simulink model "pendule_inv_echant_etu"  (R2022b)
settings: Solver=VariableStepAuto  StartTime=0.0  StopTime=10.0  RelTol=1e-3
values from neighbouring files (symbols this model uses):
  g = 9.81    [simu_pendule_inv_capteur_etu.m]    (also in simu_pendule_inv_etu.m)
  K = [10 1]    [simu_pendule_inv_capteur_etu.m]    (also in simu_pendule_inv_etu.m = [30 10])
  l = 10    [simu_pendule_inv_capteur_etu.m]    (also in simu_pendule_inv_etu.m)
  ue = 0    [simu_pendule_inv_capteur_etu.m]    (also in simu_pendule_inv_etu.m)
  x0 = [pi/20 0]'    [simu_pendule_inv_capteur_etu.m]    (also in simu_pendule_inv_etu.m = [pi/10 0]')
  xe = [0 0]'    [simu_pendule_inv_capteur_etu.m]    (also in simu_pendule_inv_etu.m)
undefined symbols (not defined in the file or in its folder): delta_t, DiscIntNeverNeededParam
settings Model: Creator=marga  LastModifiedBy=marga

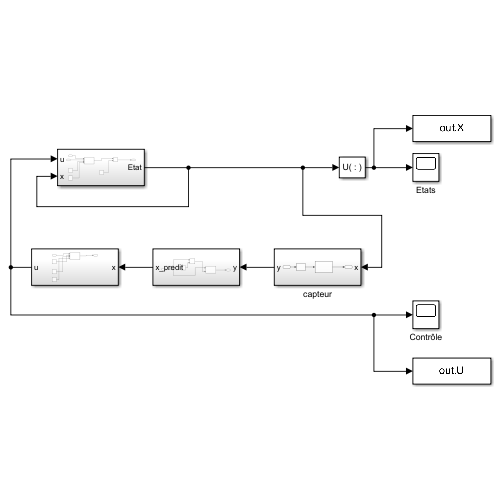
[thumbnail: Simulink's stored preview of the top-level diagram]
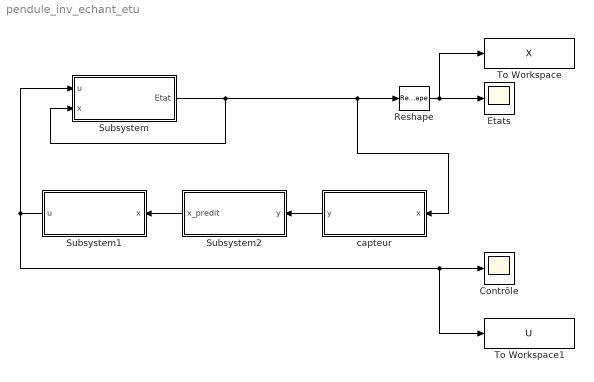
== system pendule_inv_echant_etu ==
  Contrôle : Scope
  Etats : Scope
  Reshape : Reshape
  Subsystem : Subsystem
  Subsystem1 : Subsystem
  Subsystem2 : Subsystem
  To Workspace : ToWorkspace  VariableName=X  SaveFormat=Timeseries  SampleTime=-1
  To Workspace1 : ToWorkspace  VariableName=U  SaveFormat=Timeseries  SampleTime=-1
  capteur : Subsystem
  wires:
  Subsystem2/1(x_predit) -> Subsystem1/1(x)
  capteur/1(y) -> Subsystem2/1(y)
  Reshape/1 -> To Workspace/1, Etats/1
  Subsystem/1(Etat) -> Subsystem/2(x), capteur/1(x), Reshape/1
  Subsystem1/1(u) -> Subsystem/1(u), To Workspace1/1, Contrôle/1

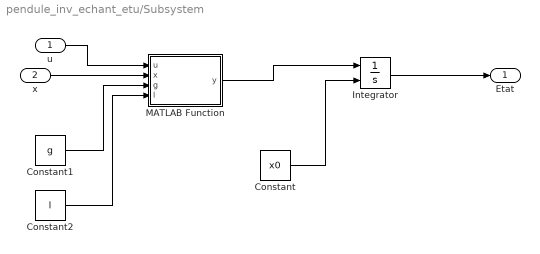
== system pendule_inv_echant_etu/Subsystem ==
  u : Inport
  x : Inport  Port=2
  Constant : Constant  Value=x0
  Constant1 : Constant  Value=g
  Constant2 : Constant  Value=l
  Integrator : Integrator  InitialConditionSource=external
  MATLAB Function : MATLAB Function  TreatAsAtomicUnit=on
  Etat : Outport
  wires:
  Constant/1 -> Integrator/2
  u/1 -> MATLAB Function/1(u)
  Integrator/1 -> Etat/1
  Constant1/1 -> MATLAB Function/3(g)
  Constant2/1 -> MATLAB Function/4(l)
  MATLAB Function/1(y) -> Integrator/1
  x/1 -> MATLAB Function/2(x)

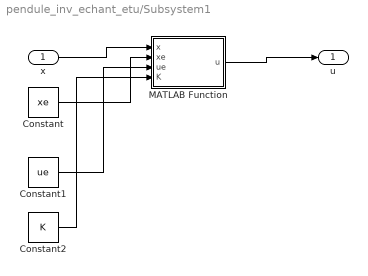
== system pendule_inv_echant_etu/Subsystem1 ==
  x : Inport
  Constant : Constant  Value=xe
  Constant1 : Constant  Value=ue
  Constant2 : Constant  Value=K  VectorParams1D=off
  MATLAB Function : MATLAB Function  TreatAsAtomicUnit=on
  u : Outport
  wires:
  x/1 -> MATLAB Function/1(x)
  MATLAB Function/1(u) -> u/1
  Constant/1 -> MATLAB Function/2(xe)
  Constant1/1 -> MATLAB Function/3(ue)
  Constant2/1 -> MATLAB Function/4(K)

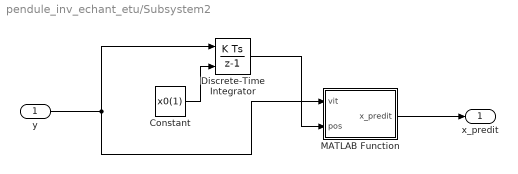
== system pendule_inv_echant_etu/Subsystem2 ==
  y : Inport
  Constant : Constant  Value=x0(1)
  Discrete-Time Integrator : DiscreteIntegrator  InitialConditionSource=external  SampleTime=delta_t  ICPrevOutput=DiscIntNeverNeededParam  ICPrevScaledInput=DiscIntNeverNeededParam
  MATLAB Function : MATLAB Function  TreatAsAtomicUnit=on
  x_predit : Outport
  wires:
  y/1 -> Discrete-Time Integrator/1, MATLAB Function/1(vit)
  Discrete-Time Integrator/1 -> MATLAB Function/2(pos)
  MATLAB Function/1(x_predit) -> x_predit/1
  Constant/1 -> Discrete-Time Integrator/2

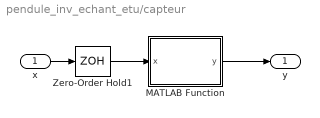
== system pendule_inv_echant_etu/capteur ==
  x : Inport
  MATLAB Function : MATLAB Function  TreatAsAtomicUnit=on
  Zero-Order Hold1 : ZeroOrderHold  SampleTime=delta_t
  y : Outport
  wires:
  x/1 -> Zero-Order Hold1/1
  MATLAB Function/1(y) -> y/1
  Zero-Order Hold1/1 -> MATLAB Function/1(x)

== matlab function pendule_inv_echant_etu/Subsystem1/MATLAB Function ==
  data: x input; u output; xe input; ue input; K input
function u = fcn(x,xe,ue,K)


u = ue + K(:)' * (x(:)-xe(:)) ;

== matlab function pendule_inv_echant_etu/Subsystem/MATLAB Function ==
  data: u input; y output; x input; g input; l input
function y = fcn(u,x,g,l)
y1 = x(2);
y2 = g / l * sin(x(1)) - cos(x(1)) * u / l;
y = [y1 y2];

== matlab function pendule_inv_echant_etu/capteur/MATLAB Function ==
  data: x input; y output
function y = fcn(x)

y = x(2);

== matlab function pendule_inv_echant_etu/Subsystem2/MATLAB Function ==
  data: vit input; x_predit output; pos input
function x_predit = fcn(vit,pos)

x_predit = [pos,vit];
